simulink model "STR"  (R2018a)
settings: Solver=ode45  StartTime=0.0  StopTime=200  RelTol=1e-3  EnableMultiTasking=on
libraries: adaptlib x1
settings Model: Creator=Administrator  LastModifiedBy=edward
settings DataIOCC: LimitDataPoints=on  SaveFormat=Array  SignalLoggingSaveFormat=ModelDataLogs
settings OptimizationCC: ExpressionDepthLimit=2147483647  InitFltsAndDblsToZero=on  LifeSpan=inf
settings DebuggingCC: SaveWithParameterizedLinksMsg=none  UnderspecifiedInitializationDetection=Classic  MergeDetectMultiDrivingBlocksExec=none  SolverPrmCheckMsg=warning  MultiTaskCondExecSysMsg=none  FcnCallInpInsideContextMsg=warning  StateNameClashWarn=warning  SFUnexpectedBacktrackingDiag=warning  SFNoUnconditionalDefaultTransitionDiag=warning  SFExecutionAtInitializationDiag=none
settings HardwareCC: ProdBitPerPointer=32  ProdBitPerSizeT=32  ProdBitPerPtrDiffT=32  ProdLargestAtomicFloat=None  ProdIntDivRoundTo=Undefined  ProdEndianess=Unspecified  ProdWordSize=32  ProdHWDeviceType=32-bit Generic
settings ModelReferenceCC: PropagateSignalLabelsOutOfModel=off
settings CodeAppCC: StateflowObjectComments=on
settings GRTTargetCC: TargetFcnLib=ansi_tfl_tmw.mat  TargetLangStandard=C89/C90 (ANSI)  GeneratePreprocessorConditionals=Disable all  CombineOutputUpdateFcns=off  GRTInterface=on
settings ConfigComp: CovMetricSettings=dw  CovHtmlReporting=on  CovSaveCumulativeToWorkspaceVar=on  CovSaveSingleToWorkspaceVar=on  CovExternalEMLEnable=off

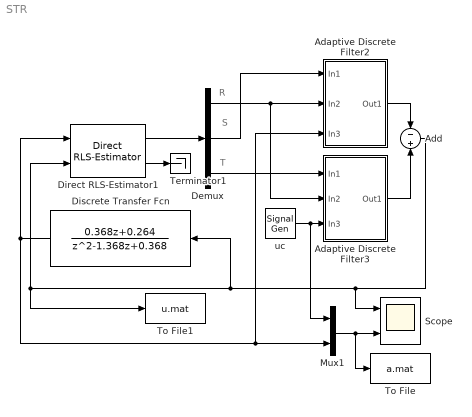
== system STR ==
  note: R
  note: S
  note: T
  Adaptive Discrete Filter2 : Subsystem  AncestorBlock=adaptlib/Adaptive Discrete Filter  mask{n_N=1, n_D=1, h=0.5}
      mask prompts: n_N "n_N (degree numerator)"; n_D "n_D (degree denominator)"
      mask Display: disp(' Num(z) \n \n Den(z) \n \n u')
  Adaptive Discrete Filter3 : Subsystem  AncestorBlock=adaptlib/Adaptive Discrete Filter  mask{n_N=1, n_D=1, h=0.5}
      mask prompts: n_N "n_N (degree numerator)"; n_D "n_D (degree denominator)"
      mask Display: disp(' Num(z) \n \n Den(z) \n \n u')
  Add : Sum  Inputs=-+
  Demux : Demux  Outputs=3
  Direct RLS-Estimator1 : adaptlib/Direct RLS-Estimator  Priority=1  n_r=1  theta_0=[1;1;-0.9;0.1]  P_0=4*eye(4)  lambda=1  A_m=[1, -1.3205,0.4966]  A_o=1  d0=1  h=0.5
  Discrete Transfer Fcn : DiscreteTransferFcn  Numerator=[0.368 0.264]  Denominator=[1 -1.368 0.368]
  Mux1 : Mux  Inputs=2
  Scope : Scope  NumInputPorts=2
  Terminator1 : Terminator
  To File : ToFile  Filename=a.mat  MatrixName=a
  To File1 : ToFile  Filename=u.mat  MatrixName=u
  uc : SignalGenerator  WaveForm=square  Amplitude=-1  Frequency=0.01
  wires:
  Direct RLS-Estimator1/2 -> Terminator1/1
  Adaptive Discrete Filter2/1(Out1) -> Add/1
  Adaptive Discrete Filter3/1(Out1) -> Add/2
  Direct RLS-Estimator1/1 -> Demux/1
  Demux/1 -> Adaptive Discrete Filter2/2(In2), Adaptive Discrete Filter3/2(In2)
  Demux/2 -> Adaptive Discrete Filter2/1(In1)
  Demux/3 -> Adaptive Discrete Filter3/1(In1)
  uc/1 -> Mux1/1, Adaptive Discrete Filter3/3(In3)
  Add/1 -> Discrete Transfer Fcn/1, Direct RLS-Estimator1/2, To File1/1, Scope/1
  Discrete Transfer Fcn/1 -> Mux1/2, Adaptive Discrete Filter2/3(In3), Direct RLS-Estimator1/1
  Mux1/1 -> To File/1, Scope/2

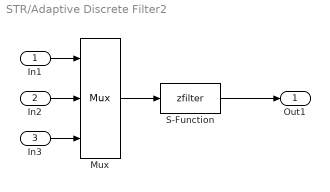
== system STR/Adaptive Discrete Filter2 ==
  In1 : Inport
  In2 : Inport  Port=2
  In3 : Inport  Port=3
  Mux : Mux  Inputs=[n_N+1 n_D+1 1]
  S-Function : S-Function  FunctionName=zfilter  Parameters=n_D,n_N,h  SFunctionDeploymentMode=off  EnableBusSupport=off
  Out1 : Outport
  wires:
  In1/1 -> Mux/1
  In2/1 -> Mux/2
  In3/1 -> Mux/3
  Mux/1 -> S-Function/1
  S-Function/1 -> Out1/1

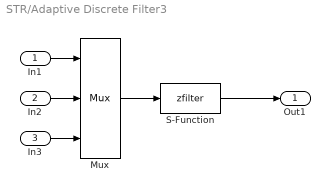
== system STR/Adaptive Discrete Filter3 ==
  In1 : Inport
  In2 : Inport  Port=2
  In3 : Inport  Port=3
  Mux : Mux  Inputs=[n_N+1 n_D+1 1]
  S-Function : S-Function  FunctionName=zfilter  Parameters=n_D,n_N,h  SFunctionDeploymentMode=off  EnableBusSupport=off
  Out1 : Outport
  wires:
  S-Function/1 -> Out1/1
  Mux/1 -> S-Function/1
  In3/1 -> Mux/3
  In2/1 -> Mux/2
  In1/1 -> Mux/1
